simulink library "Generator_Lib_org"  (Simulink 10.0)
settings: Solver=ode45  StartTime=0.0  StopTime=10.0  RelTol=1e-3  EnableMultiTasking=on
undefined symbols (not defined in the file): radps2rpm, WT_Params
libraries: powerlib x12, fl_lib x10, nesl_utility x4, $bdroot x1, powerlib_extras x1
Description:
  | Copyright 2009-2017 The MathWorks, Inc. MathWorks, Inc.
settings Model: Creator=smiller  LastModifiedBy=bhisma

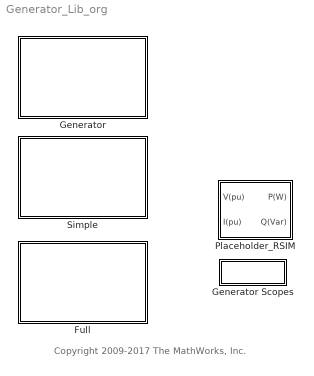
== system Generator_Lib_org ==
  note: Copyright 2009-2017 The MathWorks, Inc.
  Full : Subsystem
      mask Display:
      | image(imread('Generator_Full_IMAGE.jpg'));
      | port_label('LConn',1,'M');
      | port_label('LConn',2,'G');
      | port_label('RConn',1,'GrVa');
      | port_label('RConn',2,'GrVb');
      | port_label('RConn',3,'GrVc');
  Generator : Subsystem  BlockChoice=Full
      settings: TemplateBlock=self  MemberBlocks=Full,Simple
      mask Display: disp(' ')
  Generator Scopes : Subsystem
  Placeholder_RSIM : Subsystem
  Simple : Subsystem
      mask Display:
      | image(imread('Generator_Simple_IMAGE.jpg'));
      | port_label('LConn',1,'M');
      | port_label('LConn',2,'G');
      | port_label('RConn',1,'GrVa');
      | port_label('RConn',2,'GrVb');
      | port_label('RConn',3,'GrVc');

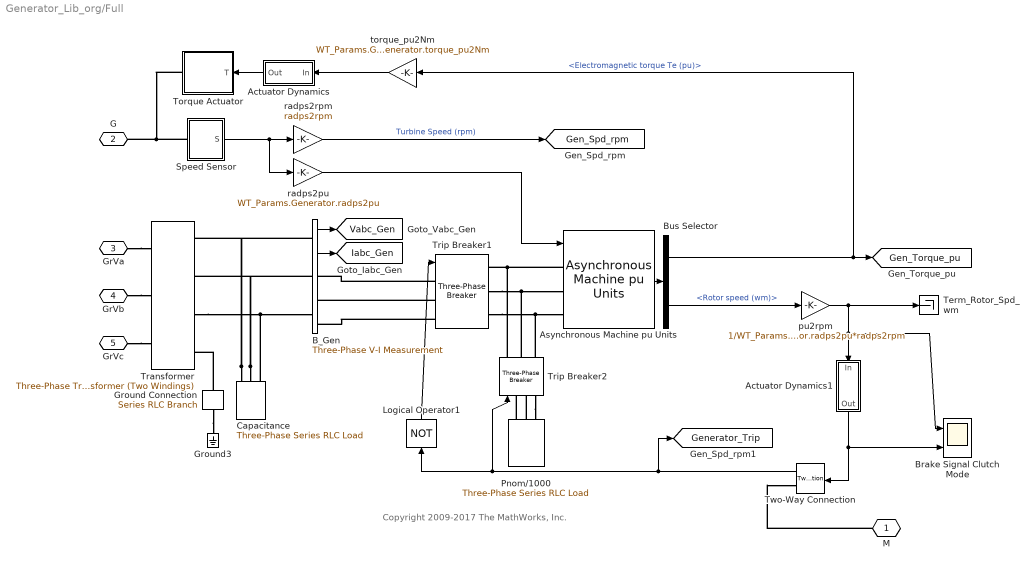
== system Generator_Lib_org/Full ==
  note: Copyright 2009-2017 The MathWorks, Inc.
  Actuator Dynamics : Subsystem  mask(First-order lag supporting vector signals){b=WT_Params.Generator.generator_time_constant, x_initial=0}
      mask prompts: b "Filter time constant"; x_initial "Initial output"
      mask help: Models a lag of the form 1/(b*s+1) where s is the Laplace operator.
  Actuator Dynamics1 : Subsystem  mask(First-order lag supporting vector signals){b=WT_Params.Generator.generator_time_constant, x_initial=0}
      mask prompts: b "Filter time constant"; x_initial "Initial output"
      mask help: Models a lag of the form 1/(b*s+1) where s is the Laplace operator.
  Asynchronous Machine pu Units : powerlib/Machines/Asynchronous Machine pu Units  RotorType=Squirrel-cage  PresetModel=No  MechanicalLoad=Speed w  ShowDetailedParameters=on  ReferenceFrame=Rotor  Units=pu  MeasurementBus=off  NominalParameters="[WT_Params.Generator.nominal_power  WT_Params.Generator.voltage WT_Params.Generator.frequency]"  Stator=[WT_Params.Generator.Stator.resistance WT_Params.Generator.Stator.inductance]  Rotor=[WT_Params.Generator.Rotor.resistance WT_Params.Generator.Rotor.inductance]  Cage1=[0.01909 0.0397]  Cage2=[0.01909 0.0397]  Lm=WT_Params.Generator.mutual_inductance  Mechanical=[0.09526 0.05479 3]  PolePairs=3  InitialConditions=[1 0 0 0 0 0 0 0]  SimulateSaturation=off  Saturation="[0.212,0.4201,0.8125,1.0979,1.4799,2.2457,3.2586,4.5763,6.4763 ;   0.5,0.7,0.9,1,1.1,1.2 ,1.3,1.4,1.5]"  LoadFlowParameters=1650000  TsPowergui=0  TsBlock=-1  IterativeModel=Forward Euler  IterativeDiscreteModel=Trapezoidal non iterative  Pmec=0
      settings: SourceProductName=Simscape Electrical  SourceProductBaseCode=PS
  B_Gen : powerlib/Measurements/Three-Phase V-I Measurement  VoltageMeasurement=phase-to-ground  SetLabelV=off  LabelV=Vabc  Vpu=on  VpuLL=off  CurrentMeasurement=yes  SetLabelI=off  LabelI=Iabc  Ipu=on  Pbase=WT_Params.Generator.nominal_power  Vbase=WT_Params.Generator.voltage  OutputType=Complex  PhasorSimulation=on  PSBequivalent=0
      settings: SourceProductName=Simscape Electrical
  Brake Signal Clutch Mode : Scope  NumInputPorts=2
  Bus Selector : BusSelector  OutputSignals=Mechanical.Electromagnetic torque Te (pu),Mechanical.Rotor speed (wm)
  Capacitance : powerlib/Elements/Three-Phase Series RLC Load  LConnTagsString=A|B|C  Configuration=Delta  NominalVoltage=WT_Params.Generator.voltage  Vabc=[1e3 1e3 1e3]  Vabcp=[1e3 1e3 1e3]  NominalFrequency=WT_Params.Generator.frequency  UnbalancedPower=off  ActivePower=0  InductivePower=0  CapacitivePower=200e3  Pabc=[10e3 9e3 11e3]  QLabc=[100 90 110]  QCabc=[100 90 110]  Pabcp=[10e3 9e3 11e3]  QLabcp=[100 90 110]  QCabcp=[100 90 110]  Measurements=None  LoadType=constant Z
      settings: SourceProductName=Simscape Electrical
  Ground Connection : powerlib/Elements/Series RLC Branch  LConnTagsString=__new0  RConnTagsString=__new0  BranchType=R  Resistance=10  Inductance=1.0  SetiL0=off  InitialCurrent=0  Capacitance=1.0  Setx0=off  InitialVoltage=0  Measurements=None
      settings: SourceProductName=Simscape Electrical
  Ground3 : powerlib/Elements/Ground  LConnTagsString=a
      settings: SourceProductName=Simscape Electrical
  Logical Operator1 : Logic  Operator=NOT  AllPortsSameDT=off  OutDataTypeStr=float('double')  SampleTime=0
  Pnom/1000 : powerlib/Elements/Three-Phase Series RLC Load  LConnTagsString=A|B|C  Configuration=Y (grounded)  NominalVoltage=WT_Params.Generator.voltage  Vabc=[1e3 1e3 1e3]  Vabcp=[1e3 1e3 1e3]  NominalFrequency=WT_Params.Generator.frequency  UnbalancedPower=off  ActivePower=WT_Params.Generator.nominal_power  InductivePower=0  CapacitivePower=0  Pabc=[10e3 9e3 11e3]  QLabc=[100 90 110]  QCabc=[100 90 110]  Pabcp=[10e3 9e3 11e3]  QLabcp=[100 90 110]  QCabcp=[100 90 110]  Measurements=None  LoadType=constant Z
      settings: SourceProductName=Simscape Electrical
  Speed Sensor : Subsystem
      mask Display:
      | plot([149.600878633536;150.016472378793;150.47508104106;150.972287968219;151.50330478576;152.063017511447;152.646035805762;153.246744883819;153.859359588817;154.477980106257;155.096648782383;155.709407499646;156.310355056631;156.893703999851;157.453836360095;157.985357756531;158.483149347555;158.942417128023;159.358738098149;159.728102859405;160.046954227227;160.312221488639;160.521349974904;160.672325664379;160.763694578642;160.794576785101;160.764674871227;160.674276808796;160.524253180566;160.316048796087;160.051668777399;159.733659248606;159.365082815313;158.949489070056;158.490880407788;157.993673480629;157.462656663088;156.908284800231], [156.971389291536;157.430657072004;157.84697804213;158.216342803387;158.535194171208;158.80046143262;159.009589918885;159.16056560836;159.251934522623;159.282816729083;159.252914815208;159.162516752777;159.012493124547;158.804288740068;158.53990872138;158.221899192587;157.853322759294;157.437729014037;156.979120351769;156.48191342461;155.950896607069;155.391183881382;154.808165587067;154.20745650901;153.594841804012;152.976221286573;152.357552610446;151.744793893183;151.143846336199;150.560497392978;150.000365032735;149.468843636298;148.971052045274;148.511784264806;148.095463294681;147.726098533424;147.407247165603;147.144199990631])
      | plot([152.057635404444;152.93604260309;153.834625296826;154.744729643097;155.657590839533;156.564417533794;157.45647648909;158.325176690034;159.162152078811;159.959342124889;160.709069452336;161.404113777147;162.037781442523;162.603969882449;163.097226392739;163.512800643557;163.846690427691;164.095680203997;164.257372064819;164.330208829146;164.313489039122;164.27939575172], [142.228020686971;141.979030910664;141.817339049842;141.744502285515;141.761222075539;141.867337399197;142.061826307913;142.342815767178;142.707599694895;143.152665022428;143.673725527376;144.265763112236;144.923076131425;145.639334301243;146.40763966397;147.220593018964;148.070365181011;148.948772379657;149.847355073393;150.757459419663;151.6703206161;152.055850472277])
      | plot([116.468514315784;116.438789536125;116.349901463023;116.202706137216;115.998621130155;115.739611892022;115.42817282337;115.067303252679;114.660478551187;114.211616663162;113.725040373958;113.205435679231;112.657806656235;112.087427271827;111.499790591278;110.900555877058;110.29549408704;109.690432297022;109.091197582803;108.503560902254;107.933181517846;107.38555249485;106.865947800123;106.379371510919;105.930509622894;105.523684921402;105.162815350711;104.851376282059;104.592367043926;104.388282036865;104.241086711057;104.152198637956;104.122473858297;104.152198637956;104.241086711057;104.388282036865;104.592367043926;104.851376282059;105.162815350711;105.523684921402;105.930509622894;106.379371510919;106.865947800123;107.38555249485;107.933181517846;108.503560902254;109.091197582803;109.690432297022;110.29549408704;110.900555877058;111.499790591278;112.087427271827;112.657806656235;113.205435679231;113.725040373958;114.211616663162;114.660478551187;115.067303252679;115.42817282337;115.739611892022;115.998621130155;116.202706137216;116.349901463023;116.438789536125;116.468514315784;116.468514315784], [111.618284136057;111.013222346039;110.413987631819;109.826350951271;109.255971566862;108.708342543866;108.188737849139;107.702161559936;107.253299671911;106.846474970419;106.485605399728;106.174166331075;105.915157092943;105.711072085881;105.563876760074;105.474988686973;105.445263907313;105.474988686973;105.563876760074;105.711072085881;105.915157092943;106.174166331075;106.485605399728;106.846474970419;107.253299671911;107.702161559936;108.188737849139;108.708342543866;109.255971566862;109.826350951271;110.413987631819;111.013222346039;111.618284136057;112.223345926075;112.822580640295;113.410217320843;113.980596705252;114.528225728247;115.047830422975;115.534406712178;115.983268600203;116.390093301695;116.750962872386;117.062401941038;117.321411179171;117.525496186232;117.67269151204;117.761579585141;117.7913043648;117.761579585141;117.67269151204;117.525496186232;117.321411179171;117.062401941038;116.750962872386;116.390093301695;115.983268600203;115.534406712178;115.047830422975;114.528225728247;113.980596705252;113.410217320843;112.822580640295;112.223345926075;111.618284136057;111.618284136057])
      | plot([239.23602886498;238.828071429858;237.608127977604;235.587947230552;232.78698463364;229.232214987837;224.957872668068;220.005121927465;214.421660463109;208.261260061133;201.583248745024;194.451939414329;186.936010476274;179.107844435155;171.042830809261;162.818640088593;154.514475725591;146.210311362589;137.986120641921;129.921107016027;122.092940974909;114.577012036853;107.445702706158;100.76769139005;94.607290988073;89.0238295237172;84.0710787831142;79.7967364633452;76.2419668175427;73.4410042206305;71.4208234735788;70.2008800213248;69.7929225862026;70.2008800213248;71.4208234735788;73.4410042206306;76.2419668175428;79.7967364633454;84.0710787831144;89.0238295237174;94.6072909880733;100.76769139005;107.445702706159;114.577012036853;122.092940974909;129.921107016027;137.986120641921;146.210311362589;154.514475725591;162.818640088593;171.042830809261;179.107844435155;186.936010476274;194.451939414329;201.583248745024;208.261260061133;214.421660463109;220.005121927465;224.957872668068;229.232214987837;232.78698463364;235.587947230552;237.608127977604;238.828071429858;239.23602886498;239.23602886498], [155.774275772274;147.47628550917;139.258209428443;131.199192095207;123.376846251889;115.866505365088;108.740498123116;102.067451871182;95.9116316925529;90.3323215006612;85.3832531026163;81.1120887325275;77.5599620381344;74.7610819412943;72.742403187363;71.5233667562631;71.1157126352191;71.5233667562631;72.742403187363;74.7610819412943;77.5599620381345;81.1120887325275;85.3832531026164;90.3323215006612;95.9116316925529;102.067451871182;108.740498123116;115.866505365089;123.376846251889;131.199192095207;139.258209428443;147.47628550917;155.774275772274;164.072266035377;172.290342116104;180.34935944934;188.171705292658;195.682046179459;202.808053421432;209.481099673365;215.636919851994;221.216230043886;226.165298441931;230.43646281202;233.988589506413;236.787469603253;238.806148357184;240.025184788284;240.432838909328;240.025184788284;238.806148357184;236.787469603253;233.988589506413;230.43646281202;226.165298441931;221.216230043886;215.636919851994;209.481099673365;202.808053421432;195.682046179459;188.171705292658;180.34935944934;172.290342116105;164.072266035378;155.774275772274;155.774275772274])
      | plot([252.715889364481;252.243022716633;250.828976737403;248.487369462568;245.240751850236;241.120390602797;236.165967051481;230.425195003451;223.953361231755;216.812793033479;209.072257983804;200.806301666664;192.094529760025;183.020841389688;173.672621134841;164.139897466795;154.514475725591;144.889053984387;135.356330316341;126.008110061494;116.934421691157;108.222649784518;99.9566934673787;92.2161584177032;85.075590219427;78.6037564477313;72.8629843997015;67.9085608483856;63.7881996009461;60.5415819886144;58.199974713779;56.7859287345493;56.3130620867014;56.7859287345493;58.1999747137791;60.5415819886146;63.7881996009463;67.9085608483858;72.8629843997018;78.6037564477315;85.0755902194273;92.2161584177035;99.9566934673791;108.222649784519;116.934421691157;126.008110061494;135.356330316341;144.889053984387;154.514475725591;164.139897466796;173.672621134841;183.020841389688;192.094529760025;200.806301666664;209.072257983803;216.812793033479;223.953361231755;230.425195003451;236.165967051481;241.120390602797;245.240751850236;248.487369462568;250.828976737403;252.243022716633;252.715889364481;252.715889364481], [154.514475725591;144.895228084285;135.36861905618;126.026395093992;116.958526921455;108.252343066071;99.9916888376535;92.2561188521535;85.1201308772245;78.6524483779929;72.9153586725213;67.9641130708855;63.8463947748555;60.6018596625959;58.2617543808809;56.8486154228053;56.3760520890355;56.8486154228053;58.2617543808809;60.6018596625959;63.8463947748555;67.9641130708856;72.9153586725213;78.652448377993;85.1201308772246;92.2561188521536;99.9916888376536;108.252343066072;116.958526921455;126.026395093992;135.36861905618;144.895228084285;154.514475725591;164.133723366898;173.660332395002;183.002556357191;192.070424529728;200.776608385111;209.037262613529;216.772832599029;223.908820573958;230.37650307319;236.113592778661;241.064838380297;245.182556676327;248.427091788587;250.767197070302;252.180336028377;252.652899362147;252.180336028377;250.767197070301;248.427091788587;245.182556676327;241.064838380297;236.113592778661;230.37650307319;223.908820573958;216.772832599029;209.037262613529;200.776608385111;192.070424529728;183.002556357191;173.660332395002;164.133723366898;154.514475725592;154.514475725591])
      | plot([154.514475725591;129.948374815285;179.017586633563;154.514475725591], [240.369848906994;203.583687543869;203.583687543869;240.369848906994])
      | plot([105.382273904979;149.60125554353], [115.271704271436;156.971085816622])
      | plot([144.688035361469;144.688035361469], [152.057865634561;203.583687543869])
      | plot([164.277926087379;164.277926087379], [152.057865634561;203.583687543869])
      | plot([159.112745895982;159.616665914655], [149.60125554353;149.60125554353])
      | plot([115.208714269102;159.364705905318], [107.901873998344;149.60125554353])
      | plot([0;311.800511553884;311.800511553884;0;0], [311.800511553884;311.800511553884;0;0;311.800511553884])
      | ;
      | color('red');
      | port_label('LConn', 1,'R')
      | port_label('output', 1,'W')
  Term_Rotor_Spd_wm : Terminator
  Torque Actuator : Subsystem
      mask Display:
      | plot([198.657636314574;187.5372000791;176.524559560751;165.725772507838;155.244837142898;145.182690602959;135.636236859729;126.697413481378;118.452306223496;110.980319976212;104.353414051689;98.6354091766174;93.8813728637222;90.1370890815176;87.4386173296598;85.811945366254;85.272738931537;85.8261908782356;87.4669711615554;90.1792781704262;93.9369909056548;98.7039205394262;104.434158933498;111.072520759669;118.555074964656;126.809760461083;135.75708011515;145.310866347487;155.379110974044;165.864851295207;176.667103899592;187.681837189509;192.988368326926], [283.691199740558;283.13774779386;281.49696751054;278.784660501669;275.026947766441;270.260018132669;264.529779738597;257.891417912426;250.40886370744;242.154178211013;233.206858556945;223.653072324609;213.584827698051;203.099087376889;192.296834772503;181.282101482586;170.160965409986;159.040529174513;148.027888656163;137.22910160325;126.748166238311;116.686019698372;107.139565955142;98.2007425767901;89.9556353189084;82.4836490716241;75.8567431471018;70.1387382720299;65.3847019591348;61.6404181769301;58.9419464250722;57.3152744616664;56.9214337615639])
      | plot([85.209725657478;1.11807254143059;1.11807254143059], [170.435198815539;170.435198815539;171.380048850551])
      | plot([283.691223012283;397.073227213696], [170.309218810871;170.309218810871])
      | plot([153.301918180659;255.34572196193], [170.309218810871;170.309218810871])
      | plot([198.654719861224;113.618216710165;198.654719861224], [85.2727156598121;170.309218810871;255.34572196193])
      | plot([198.654719861224;153.301918180659;198.654719861224], [215.662020491436;170.309218810871;124.956417130306])
      | plot([198.654719861224;283.691223012283;283.691223012283;187.316519441083;192.985619651154], [283.691223012283;283.691223012283;56.927214609459;56.927214609459;56.927214609459])
      | 
      | patch([395.419739652425;395.419739652425;5.6843418860808e-14;0;395.419739652425;394.947314634919;0.472425017505884;0.472425017505941;394.947314634919;394.947314634919;395.419739652425], [340.618437621742;5.6843418860808e-14;0;340.618437621742;340.618437621742;340.146012604237;340.146012604237;0.472425017505884;0.472425017505884;340.146012604237;340.618437621742], [1;1;1])
      | ;
      | color('red');
      | port_label('RConn', 1,'R')
      | port_label('Input', 1,'T')
  Transformer : powerlib/Elements/Three-Phase Transformer (Two Windings)  Winding1Connection=Yg  Winding2Connection=Yn  CoreType=Three single-phase transformers  SetSaturation=off  Hysteresis=off  DataFile='hysteresis'  SetInitialFlux=off  Measurements=None  UNITS=pu  NominalPower="[2e6  60]"  Winding1=[WT_Params.Grid.voltage, 0.025/30 , 0.025]  Winding2=[ WT_Params.Generator.voltage, 0.025/30 , 0.025]  Rm=500  Lm=inf  L0=0.5  Saturation=[ 0,0 ; 0.0024,1.2 ; 1.0,1.52 ]  InitialFluxes=[ 0.8 , -0.8 , 0.7 ]  BreakLoop=off  DiscreteSolver=Trapezoidal iterative  DataType=off  TransfoNumber=0
      settings: SourceProductName=Simscape Electrical
  Trip Breaker1 : powerlib/Elements/Three-Phase Breaker  InitialState=closed  SwitchA=on  SwitchB=on  SwitchC=on  SwitchTimes="[4/60  10/60]"  External=on  BreakerResistance=WT_Params.Generator.Breakers.ron  SnubberResistance=WT_Params.Generator.Breakers.rp  SnubberCapacitance=WT_Params.Generator.Breakers.cp  Measurements=None
      settings: SourceProductName=Simscape Electrical
  Trip Breaker2 : powerlib/Elements/Three-Phase Breaker  InitialState=open  SwitchA=on  SwitchB=on  SwitchC=on  SwitchTimes="[4/60  10/60]"  External=on  BreakerResistance=WT_Params.Generator.Breakers.ron  SnubberResistance=WT_Params.Generator.Breakers.rp  SnubberCapacitance=WT_Params.Generator.Breakers.cp  Measurements=None
      settings: SourceProductName=Simscape Electrical
  Two-Way Connection : TwoWayConnection
  pu2rpm : Gain  Gain=1/WT_Params.Generator.radps2pu*radps2rpm
  radps2pu : Gain  Gain=WT_Params.Generator.radps2pu
  radps2rpm : Gain  Gain=radps2rpm
  torque_pu2Nm : Gain  Gain=WT_Params.Generator.torque_pu2Nm
  M : PMIOPort  Tag=PMCPort  Side=Left
  G : PMIOPort  Port=2  Side=Left
  GrVa : PMIOPort  Port=3  Side=Right
  GrVb : PMIOPort  Port=4  Side=Right
  GrVc : PMIOPort  Port=5  Side=Right
  tag scope: Gen_Spd_rpm=global, Gen_Torque_pu=global, Generator_Trip=global, Iabc_Gen=global, Vabc_Gen=global
  wires:
  Logical Operator1/1 -> Trip Breaker1/1
  Two-Way Connection/1 -> Logical Operator1/1, Trip Breaker2/1, [Generator_Trip]
  pu2rpm/1 -> Brake Signal Clutch Mode/1, Actuator Dynamics1/1(In), Term_Rotor_Spd_wm/1
  Bus Selector/2 -> pu2rpm/1  "<Rotor speed (wm)>"
  radps2rpm/1 -> [Gen_Spd_rpm]  "Turbine Speed (rpm)"
  torque_pu2Nm/1 -> Actuator Dynamics/1(In)
  radps2pu/1 -> Asynchronous Machine pu Units/1
  Bus Selector/1 -> [Gen_Torque_pu], torque_pu2Nm/1  "<Electromagnetic torque Te (pu)>"
  Speed Sensor/1(S) -> radps2pu/1, radps2rpm/1
  Asynchronous Machine pu Units/1 -> Bus Selector/1
  B_Gen/1 -> [Vabc_Gen]
  B_Gen/2 -> [Iabc_Gen]
  Actuator Dynamics/1(Out) -> Torque Actuator/1(T)
  Actuator Dynamics1/1(Out) -> Brake Signal Clutch Mode/2, Two-Way Connection/1
  connections:
  Trip Breaker1/LConn1 -- B_Gen/RConn1
  Trip Breaker1/LConn2 -- B_Gen/RConn2
  Trip Breaker1/LConn3 -- B_Gen/RConn3
  Trip Breaker2/RConn1 -- Trip Breaker1/RConn1 -- Asynchronous Machine pu Units/LConn1
  Trip Breaker2/RConn2 -- Asynchronous Machine pu Units/LConn2 -- Trip Breaker1/RConn2
  Trip Breaker2/RConn3 -- Asynchronous Machine pu Units/LConn3 -- Trip Breaker1/RConn3
  Pnom/1000/LConn2 -- Trip Breaker2/LConn2
  Trip Breaker2/LConn3 -- Pnom/1000/LConn3
  Pnom/1000/LConn1 -- Trip Breaker2/LConn1
  Ground Connection/LConn1 -- Transformer/RConn4
  Ground Connection/RConn1 -- Ground3/LConn1
  GrVa/RConn1 -- Transformer/LConn1
  GrVc/RConn1 -- Transformer/LConn3
  GrVb/RConn1 -- Transformer/LConn2
  Torque Actuator/RConn1 -- G/RConn1 -- Speed Sensor/LConn1
  Capacitance/LConn3 -- B_Gen/LConn3 -- Transformer/RConn3
  Capacitance/LConn1 -- B_Gen/LConn1 -- Transformer/RConn1
  M/RConn1 -- Two-Way Connection/RConn1
  Capacitance/LConn2 -- B_Gen/LConn2 -- Transformer/RConn2

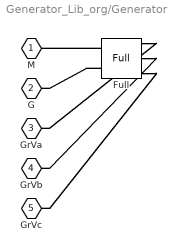
== system Generator_Lib_org/Generator ==
  Full : $bdroot/Full  SystemSampleTime=-1  Latency=0  AutoFrameSizeCalculation=off
  M : PMIOPort  Side=Left
  G : PMIOPort  Port=2  Side=Left
  GrVa : PMIOPort  Port=3  Side=Right
  GrVb : PMIOPort  Port=4  Side=Right
  GrVc : PMIOPort  Port=5  Side=Right
  connections:
  Full/LConn1 -- M/RConn1
  Full/LConn2 -- G/RConn1
  Full/RConn1 -- GrVa/RConn1
  Full/RConn2 -- GrVb/RConn1
  Full/RConn3 -- GrVc/RConn1

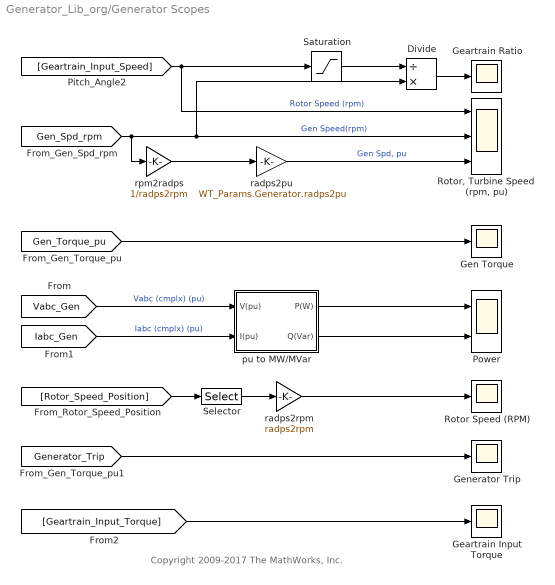
== system Generator_Lib_org/Generator Scopes ==
  note: Copyright 2009-2017 The MathWorks, Inc.
  Divide : Product  Inputs=/*
  Geartrain Input Torque : Scope
  Geartrain Ratio : Scope
  Gen Torque : Scope
  Generator Trip : Scope
  Power : Scope  NumInputPorts=2
  Rotor Speed (RPM) : Scope
  "Rotor, Turbine Speed  (rpm, pu)" : Scope  NumInputPorts=3
  Saturation : Saturate  UpperLimit=inf  LowerLimit=eps
  Selector : Selector  InputPortWidth=2  IndexOptions=Index vector (dialog)  Indices=[2]  OutputSizes=1
  pu to MW/MVar : Subsystem
  radps2pu : Gain  Gain=WT_Params.Generator.radps2pu
  radps2rpm : Gain  Gain=radps2rpm
  rpm2radps : Gain  Gain=1/radps2rpm
  wires:
  [Geartrain_Input_Torque] -> Geartrain Input Torque/1
  Saturation/1 -> Divide/1
  radps2rpm/1 -> Rotor Speed (RPM)/1
  Selector/1 -> radps2rpm/1
  [Rotor_Speed_Position] -> Selector/1
  [Gen_Spd_rpm] -> rpm2radps/1, Divide/2, "Rotor, Turbine Speed  (rpm, pu)"/2  "Gen Speed(rpm)"
  Divide/1 -> Geartrain Ratio/1
  rpm2radps/1 -> radps2pu/1
  radps2pu/1 -> "Rotor, Turbine Speed  (rpm, pu)"/3  "Gen Spd, pu"
  [Geartrain_Input_Speed] -> Saturation/1, "Rotor, Turbine Speed  (rpm, pu)"/1  "Rotor Speed (rpm)"
  [Vabc_Gen] -> pu to MW/MVar/1(V(pu))  "Vabc (cmplx) (pu)"
  [Iabc_Gen] -> pu to MW/MVar/2(I(pu))  "Iabc (cmplx) (pu)"
  [Gen_Torque_pu] -> Gen Torque/1
  pu to MW/MVar/1(P(W)) -> Power/1
  pu to MW/MVar/2(Q(Var)) -> Power/2
  [Generator_Trip] -> Generator Trip/1

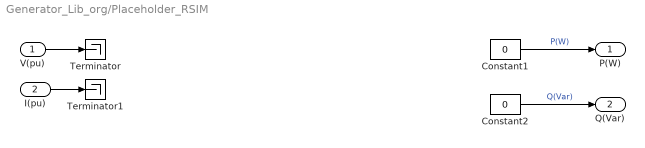
== system Generator_Lib_org/Placeholder_RSIM ==
  V(pu) : Inport
  I(pu) : Inport  Port=2
  Constant1 : Constant  Value=0
  Constant2 : Constant  Value=0
  Terminator : Terminator
  Terminator1 : Terminator
  P(W) : Outport
  Q(Var) : Outport  Port=2
  wires:
  Constant2/1 -> Q(Var)/1  "Q(Var)"
  Constant1/1 -> P(W)/1  "P(W)"
  I(pu)/1 -> Terminator1/1
  V(pu)/1 -> Terminator/1

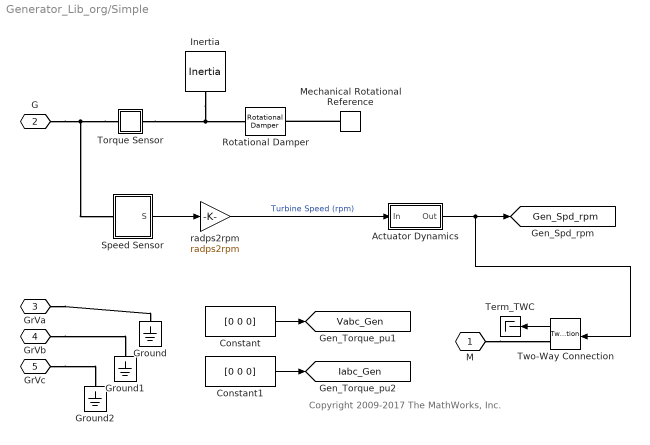
== system Generator_Lib_org/Simple ==
  note: Copyright 2009-2017 The MathWorks, Inc.
  Actuator Dynamics : Subsystem  mask(First-order lag supporting vector signals){b=WT_Params.Generator.generator_time_constant, x_initial=0}
      mask prompts: b "Filter time constant"; x_initial "Initial output"
      mask help: Models a lag of the form 1/(b*s+1) where s is the Laplace operator.
  Constant : Constant  Value=[0 0 0]  OutDataTypeStr=Inherit: Inherit via back propagation
  Constant1 : Constant  Value=[0 0 0]  OutDataTypeStr=Inherit: Inherit via back propagation
  Ground : powerlib/Elements/Ground  LConnTagsString=a
      settings: SourceProductName=Simscape Electrical
  Ground1 : powerlib/Elements/Ground  LConnTagsString=a
      settings: SourceProductName=Simscape Electrical
  Ground2 : powerlib/Elements/Ground  LConnTagsString=a
      settings: SourceProductName=Simscape Electrical
  Inertia : fl_lib/Mechanical/Rotational Elements/Inertia  inertia=WT_Params.Generator.Simple.inertia kg*m^2  w_specify=on  w_priority=High  w=0 rad/s  w_nominal_specify=off  w_nominal_unit=rad/s  w_nominal_value=1  t_specify=off  t_priority=High  t=0 N*m  t_nominal_specify=off  t_nominal_unit=N*m  t_nominal_value=1
  Mechanical Rotational Reference : fl_lib/Mechanical/Rotational Elements/Mechanical Rotational Reference
  Rotational Damper : fl_lib/Mechanical/Rotational Elements/Rotational Damper  D=WT_Params.Generator.Simple.damping N*m/(rad/s)  w_specify=off  w_priority=High  w=0 rad/s  w_nominal_specify=off  w_nominal_unit=rad/s  w_nominal_value=1  t_specify=off  t_priority=High  t=0 N*m  t_nominal_specify=off  t_nominal_unit=N*m  t_nominal_value=1
  Speed Sensor : Subsystem
      mask Display:
      | plot([149.600878633536;150.016472378793;150.47508104106;150.972287968219;151.50330478576;152.063017511447;152.646035805762;153.246744883819;153.859359588817;154.477980106257;155.096648782383;155.709407499646;156.310355056631;156.893703999851;157.453836360095;157.985357756531;158.483149347555;158.942417128023;159.358738098149;159.728102859405;160.046954227227;160.312221488639;160.521349974904;160.672325664379;160.763694578642;160.794576785101;160.764674871227;160.674276808796;160.524253180566;160.316048796087;160.051668777399;159.733659248606;159.365082815313;158.949489070056;158.490880407788;157.993673480629;157.462656663088;156.908284800231], [156.971389291536;157.430657072004;157.84697804213;158.216342803387;158.535194171208;158.80046143262;159.009589918885;159.16056560836;159.251934522623;159.282816729083;159.252914815208;159.162516752777;159.012493124547;158.804288740068;158.53990872138;158.221899192587;157.853322759294;157.437729014037;156.979120351769;156.48191342461;155.950896607069;155.391183881382;154.808165587067;154.20745650901;153.594841804012;152.976221286573;152.357552610446;151.744793893183;151.143846336199;150.560497392978;150.000365032735;149.468843636298;148.971052045274;148.511784264806;148.095463294681;147.726098533424;147.407247165603;147.144199990631])
      | plot([152.057635404444;152.93604260309;153.834625296826;154.744729643097;155.657590839533;156.564417533794;157.45647648909;158.325176690034;159.162152078811;159.959342124889;160.709069452336;161.404113777147;162.037781442523;162.603969882449;163.097226392739;163.512800643557;163.846690427691;164.095680203997;164.257372064819;164.330208829146;164.313489039122;164.27939575172], [142.228020686971;141.979030910664;141.817339049842;141.744502285515;141.761222075539;141.867337399197;142.061826307913;142.342815767178;142.707599694895;143.152665022428;143.673725527376;144.265763112236;144.923076131425;145.639334301243;146.40763966397;147.220593018964;148.070365181011;148.948772379657;149.847355073393;150.757459419663;151.6703206161;152.055850472277])
      | plot([116.468514315784;116.438789536125;116.349901463023;116.202706137216;115.998621130155;115.739611892022;115.42817282337;115.067303252679;114.660478551187;114.211616663162;113.725040373958;113.205435679231;112.657806656235;112.087427271827;111.499790591278;110.900555877058;110.29549408704;109.690432297022;109.091197582803;108.503560902254;107.933181517846;107.38555249485;106.865947800123;106.379371510919;105.930509622894;105.523684921402;105.162815350711;104.851376282059;104.592367043926;104.388282036865;104.241086711057;104.152198637956;104.122473858297;104.152198637956;104.241086711057;104.388282036865;104.592367043926;104.851376282059;105.162815350711;105.523684921402;105.930509622894;106.379371510919;106.865947800123;107.38555249485;107.933181517846;108.503560902254;109.091197582803;109.690432297022;110.29549408704;110.900555877058;111.499790591278;112.087427271827;112.657806656235;113.205435679231;113.725040373958;114.211616663162;114.660478551187;115.067303252679;115.42817282337;115.739611892022;115.998621130155;116.202706137216;116.349901463023;116.438789536125;116.468514315784;116.468514315784], [111.618284136057;111.013222346039;110.413987631819;109.826350951271;109.255971566862;108.708342543866;108.188737849139;107.702161559936;107.253299671911;106.846474970419;106.485605399728;106.174166331075;105.915157092943;105.711072085881;105.563876760074;105.474988686973;105.445263907313;105.474988686973;105.563876760074;105.711072085881;105.915157092943;106.174166331075;106.485605399728;106.846474970419;107.253299671911;107.702161559936;108.188737849139;108.708342543866;109.255971566862;109.826350951271;110.413987631819;111.013222346039;111.618284136057;112.223345926075;112.822580640295;113.410217320843;113.980596705252;114.528225728247;115.047830422975;115.534406712178;115.983268600203;116.390093301695;116.750962872386;117.062401941038;117.321411179171;117.525496186232;117.67269151204;117.761579585141;117.7913043648;117.761579585141;117.67269151204;117.525496186232;117.321411179171;117.062401941038;116.750962872386;116.390093301695;115.983268600203;115.534406712178;115.047830422975;114.528225728247;113.980596705252;113.410217320843;112.822580640295;112.223345926075;111.618284136057;111.618284136057])
      | plot([239.23602886498;238.828071429858;237.608127977604;235.587947230552;232.78698463364;229.232214987837;224.957872668068;220.005121927465;214.421660463109;208.261260061133;201.583248745024;194.451939414329;186.936010476274;179.107844435155;171.042830809261;162.818640088593;154.514475725591;146.210311362589;137.986120641921;129.921107016027;122.092940974909;114.577012036853;107.445702706158;100.76769139005;94.607290988073;89.0238295237172;84.0710787831142;79.7967364633452;76.2419668175427;73.4410042206305;71.4208234735788;70.2008800213248;69.7929225862026;70.2008800213248;71.4208234735788;73.4410042206306;76.2419668175428;79.7967364633454;84.0710787831144;89.0238295237174;94.6072909880733;100.76769139005;107.445702706159;114.577012036853;122.092940974909;129.921107016027;137.986120641921;146.210311362589;154.514475725591;162.818640088593;171.042830809261;179.107844435155;186.936010476274;194.451939414329;201.583248745024;208.261260061133;214.421660463109;220.005121927465;224.957872668068;229.232214987837;232.78698463364;235.587947230552;237.608127977604;238.828071429858;239.23602886498;239.23602886498], [155.774275772274;147.47628550917;139.258209428443;131.199192095207;123.376846251889;115.866505365088;108.740498123116;102.067451871182;95.9116316925529;90.3323215006612;85.3832531026163;81.1120887325275;77.5599620381344;74.7610819412943;72.742403187363;71.5233667562631;71.1157126352191;71.5233667562631;72.742403187363;74.7610819412943;77.5599620381345;81.1120887325275;85.3832531026164;90.3323215006612;95.9116316925529;102.067451871182;108.740498123116;115.866505365089;123.376846251889;131.199192095207;139.258209428443;147.47628550917;155.774275772274;164.072266035377;172.290342116104;180.34935944934;188.171705292658;195.682046179459;202.808053421432;209.481099673365;215.636919851994;221.216230043886;226.165298441931;230.43646281202;233.988589506413;236.787469603253;238.806148357184;240.025184788284;240.432838909328;240.025184788284;238.806148357184;236.787469603253;233.988589506413;230.43646281202;226.165298441931;221.216230043886;215.636919851994;209.481099673365;202.808053421432;195.682046179459;188.171705292658;180.34935944934;172.290342116105;164.072266035378;155.774275772274;155.774275772274])
      | plot([252.715889364481;252.243022716633;250.828976737403;248.487369462568;245.240751850236;241.120390602797;236.165967051481;230.425195003451;223.953361231755;216.812793033479;209.072257983804;200.806301666664;192.094529760025;183.020841389688;173.672621134841;164.139897466795;154.514475725591;144.889053984387;135.356330316341;126.008110061494;116.934421691157;108.222649784518;99.9566934673787;92.2161584177032;85.075590219427;78.6037564477313;72.8629843997015;67.9085608483856;63.7881996009461;60.5415819886144;58.199974713779;56.7859287345493;56.3130620867014;56.7859287345493;58.1999747137791;60.5415819886146;63.7881996009463;67.9085608483858;72.8629843997018;78.6037564477315;85.0755902194273;92.2161584177035;99.9566934673791;108.222649784519;116.934421691157;126.008110061494;135.356330316341;144.889053984387;154.514475725591;164.139897466796;173.672621134841;183.020841389688;192.094529760025;200.806301666664;209.072257983803;216.812793033479;223.953361231755;230.425195003451;236.165967051481;241.120390602797;245.240751850236;248.487369462568;250.828976737403;252.243022716633;252.715889364481;252.715889364481], [154.514475725591;144.895228084285;135.36861905618;126.026395093992;116.958526921455;108.252343066071;99.9916888376535;92.2561188521535;85.1201308772245;78.6524483779929;72.9153586725213;67.9641130708855;63.8463947748555;60.6018596625959;58.2617543808809;56.8486154228053;56.3760520890355;56.8486154228053;58.2617543808809;60.6018596625959;63.8463947748555;67.9641130708856;72.9153586725213;78.652448377993;85.1201308772246;92.2561188521536;99.9916888376536;108.252343066072;116.958526921455;126.026395093992;135.36861905618;144.895228084285;154.514475725591;164.133723366898;173.660332395002;183.002556357191;192.070424529728;200.776608385111;209.037262613529;216.772832599029;223.908820573958;230.37650307319;236.113592778661;241.064838380297;245.182556676327;248.427091788587;250.767197070302;252.180336028377;252.652899362147;252.180336028377;250.767197070301;248.427091788587;245.182556676327;241.064838380297;236.113592778661;230.37650307319;223.908820573958;216.772832599029;209.037262613529;200.776608385111;192.070424529728;183.002556357191;173.660332395002;164.133723366898;154.514475725592;154.514475725591])
      | plot([154.514475725591;129.948374815285;179.017586633563;154.514475725591], [240.369848906994;203.583687543869;203.583687543869;240.369848906994])
      | plot([105.382273904979;149.60125554353], [115.271704271436;156.971085816622])
      | plot([144.688035361469;144.688035361469], [152.057865634561;203.583687543869])
      | plot([164.277926087379;164.277926087379], [152.057865634561;203.583687543869])
      | plot([159.112745895982;159.616665914655], [149.60125554353;149.60125554353])
      | plot([115.208714269102;159.364705905318], [107.901873998344;149.60125554353])
      | plot([0;311.800511553884;311.800511553884;0;0], [311.800511553884;311.800511553884;0;0;311.800511553884])
      | ;
      | color('red');
      | port_label('LConn', 1,'R')
      | port_label('output', 1,'W')
  Term_TWC : Terminator
  Torque Sensor : Subsystem
      mask Display: disp('S');
  Two-Way Connection : TwoWayConnection
  radps2rpm : Gain  Gain=radps2rpm
  M : PMIOPort  Tag=PMCPort  Side=Left
  G : PMIOPort  Port=2  Side=Left
  GrVa : PMIOPort  Port=3  Side=Right
  GrVb : PMIOPort  Port=4  Side=Right
  GrVc : PMIOPort  Port=5  Side=Right
  tag scope: Gen_Spd_rpm=global, Iabc_Gen=global, Vabc_Gen=global
  wires:
  Constant1/1 -> [Iabc_Gen]
  Constant/1 -> [Vabc_Gen]
  Speed Sensor/1(S) -> radps2rpm/1
  radps2rpm/1 -> Actuator Dynamics/1(In)  "Turbine Speed (rpm)"
  Two-Way Connection/1 -> Term_TWC/1
  Actuator Dynamics/1(Out) -> Two-Way Connection/1, [Gen_Spd_rpm]
  connections:
  M/RConn1 -- Two-Way Connection/RConn1
  Torque Sensor/LConn1 -- G/RConn1 -- Speed Sensor/LConn1
  GrVb/RConn1 -- Ground1/LConn1
  GrVc/RConn1 -- Ground2/LConn1
  GrVa/RConn1 -- Ground/LConn1
  Mechanical Rotational Reference/LConn1 -- Rotational Damper/RConn1
  Torque Sensor/RConn1 -- Inertia/LConn1 -- Rotational Damper/LConn1

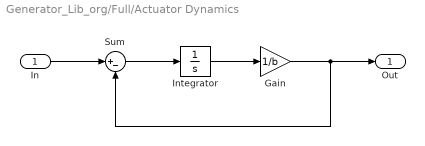
== system Generator_Lib_org/Full/Actuator Dynamics ==
  In : Inport
  Gain : Gain  Gain=1/b
  Integrator : Integrator  InitialCondition=x_initial
  Sum : Sum  Inputs=|+-  SaturateOnIntegerOverflow=on  InputSameDT=on  OutDataTypeStr=Inherit: Same as first input
  Out : Outport
  wires:
  Gain/1 -> Out/1, Sum/2
  Integrator/1 -> Gain/1
  In/1 -> Sum/1
  Sum/1 -> Integrator/1

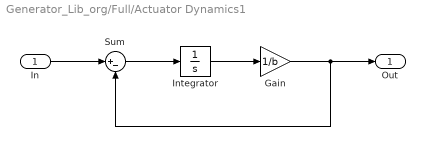
== system Generator_Lib_org/Full/Actuator Dynamics1 ==
  In : Inport
  Gain : Gain  Gain=1/b
  Integrator : Integrator  InitialCondition=x_initial
  Sum : Sum  Inputs=|+-  SaturateOnIntegerOverflow=on  InputSameDT=on  OutDataTypeStr=Inherit: Same as first input
  Out : Outport
  wires:
  Sum/1 -> Integrator/1
  In/1 -> Sum/1
  Integrator/1 -> Gain/1
  Gain/1 -> Sum/2, Out/1

== system Generator_Lib_org/Full/Speed Sensor ==
  Ideal Rotational Motion Sensor : fl_lib/Mechanical/Mechanical Sensors/Ideal Rotational Motion Sensor  offset=0 rad
  Mechanical Rotational Reference1 : fl_lib/Mechanical/Rotational Elements/Mechanical Rotational Reference
  PS-Simulink Converter : nesl_utility/PS-Simulink Converter  PhysicalDomain=network_engine_domain  SubClassName=ps_output  LeftPortType=input  RightPortType=output  PseudoPeriodic=off  Frequencies=[]  Unit=rad/s  AffineConversion=off
  R : PMIOPort  Side=Left
  S : Outport
  wires:
  PS-Simulink Converter/1 -> S/1
  connections:
  Ideal Rotational Motion Sensor/RConn2 -- PS-Simulink Converter/LConn1
  R/RConn1 -- Ideal Rotational Motion Sensor/LConn1
  Mechanical Rotational Reference1/LConn1 -- Ideal Rotational Motion Sensor/RConn1

== system Generator_Lib_org/Full/Torque Actuator ==
  T : Inport
  Ideal Torque Source : fl_lib/Mechanical/Mechanical Sources/Ideal Torque Source
  Mechanical Rotational Reference : fl_lib/Mechanical/Rotational Elements/Mechanical Rotational Reference
  Simulink-PS Converter : nesl_utility/Simulink-PS Converter  PhysicalDomain=network_engine_domain  SubClassName=ps_input  LeftPortType=input  RightPortType=output  PseudoPeriodic=off  Frequencies=[]  NoiseDistribution=none  NoiseParameters=[]  Unit=1  AffineConversion=off  FilteringAndDerivatives=filter  SimscapeFilterOrder=1  InputFilterTimeConstant=WT_Params.Generator.PSLD_Interface_Filter_Coeff  UdotUserProvided=1
  R : PMIOPort  Side=Right
  wires:
  T/1 -> Simulink-PS Converter/1
  connections:
  Simulink-PS Converter/RConn1 -- Ideal Torque Source/RConn1
  Mechanical Rotational Reference/LConn1 -- Ideal Torque Source/RConn2
  R/RConn1 -- Ideal Torque Source/LConn1

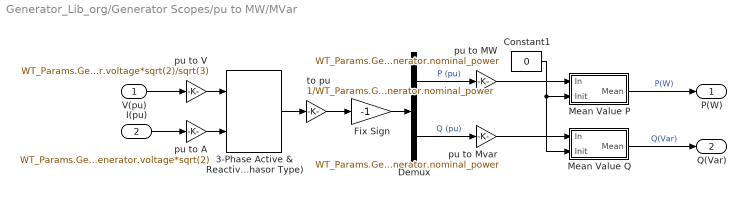
== system Generator_Lib_org/Generator Scopes/pu to MW/MVar ==
  V(pu) : Inport
  I(pu) : Inport  Port=2
  3-Phase Active & Reactive Power (Phasor Type) : powerlib_extras/Phasor Library/3-Phase Active & Reactive Power (Phasor Type)
      settings: SourceProductName=Simscape Electrical  SourceProductBaseCode=PS
  Constant1 : Constant  Value=0
  Demux : Demux  Outputs=2
  Fix Sign : Gain  Gain=-1  SaturateOnIntegerOverflow=on  OutDataTypeStr=Inherit: Same as input  ParamDataTypeStr=Inherit: Same as input
  Mean Value P : Subsystem  mask(Mean value){Period=1/WT_Params.Generator.frequency}
      mask prompts: Period "Averaging period (s):"
      mask help: This block uses the running window averaging technique to compute the mean value of the input signal over the specified period.
  Mean Value Q : Subsystem  mask(Mean value){Period=1/WT_Params.Generator.frequency}
      mask prompts: Period "Averaging period (s):"
      mask help: This block uses the running window averaging technique to compute the mean value of the input signal over the specified period.
  pu to A : Gain  Gain=WT_Params.Generator.nominal_power/sqrt(3)/WT_Params.Generator.voltage*sqrt(2)  SaturateOnIntegerOverflow=on  OutDataTypeStr=Inherit: Same as input  ParamDataTypeStr=Inherit: Same as input
  pu to MW : Gain  Gain=WT_Params.Generator.nominal_power  SaturateOnIntegerOverflow=on  OutDataTypeStr=Inherit: Same as input  ParamDataTypeStr=Inherit: Same as input
  pu to Mvar : Gain  Gain=WT_Params.Generator.nominal_power  SaturateOnIntegerOverflow=on  OutDataTypeStr=Inherit: Same as input  ParamDataTypeStr=Inherit: Same as input
  pu to V : Gain  Gain=WT_Params.Generator.voltage*sqrt(2)/sqrt(3)  SaturateOnIntegerOverflow=on  OutDataTypeStr=Inherit: Same as input  ParamDataTypeStr=Inherit: Same as input
  to pu : Gain  Gain=1/WT_Params.Generator.nominal_power  SaturateOnIntegerOverflow=on  OutDataTypeStr=Inherit: Same as input  ParamDataTypeStr=Inherit: Same as input
  P(W) : Outport
  Q(Var) : Outport  Port=2
  wires:
  Demux/1 -> pu to MW/1  "P (pu)"
  Demux/2 -> pu to Mvar/1  "Q (pu)"
  pu to V/1 -> 3-Phase Active & Reactive Power (Phasor Type)/1
  3-Phase Active & Reactive Power (Phasor Type)/1 -> to pu/1
  to pu/1 -> Fix Sign/1
  Fix Sign/1 -> Demux/1
  pu to A/1 -> 3-Phase Active & Reactive Power (Phasor Type)/2
  pu to MW/1 -> Mean Value P/1(In)
  Constant1/1 -> Mean Value P/2(Init), Mean Value Q/2(Init)
  pu to Mvar/1 -> Mean Value Q/1(In)
  V(pu)/1 -> pu to V/1
  I(pu)/1 -> pu to A/1
  Mean Value P/1(Mean) -> P(W)/1  "P(W)"
  Mean Value Q/1(Mean) -> Q(Var)/1  "Q(Var)"

== system Generator_Lib_org/Simple/Actuator Dynamics ==
  In : Inport
  Gain : Gain  Gain=1/b
  Integrator : Integrator  InitialCondition=x_initial
  Sum : Sum  Inputs=|+-  SaturateOnIntegerOverflow=on  InputSameDT=on  OutDataTypeStr=Inherit: Same as first input
  Out : Outport
  wires:
  Sum/1 -> Integrator/1
  In/1 -> Sum/1
  Integrator/1 -> Gain/1
  Gain/1 -> Sum/2, Out/1

== system Generator_Lib_org/Simple/Speed Sensor ==
  Ideal Rotational Motion Sensor : fl_lib/Mechanical/Mechanical Sensors/Ideal Rotational Motion Sensor  offset=0 rad
  Mechanical Rotational Reference1 : fl_lib/Mechanical/Rotational Elements/Mechanical Rotational Reference
  PS-Simulink Converter : nesl_utility/PS-Simulink Converter  PhysicalDomain=network_engine_domain  SubClassName=ps_output  LeftPortType=input  RightPortType=output  PseudoPeriodic=off  Frequencies=[]  Unit=1  AffineConversion=off
  R : PMIOPort  Side=Left
  S : Outport
  wires:
  PS-Simulink Converter/1 -> S/1
  connections:
  Mechanical Rotational Reference1/LConn1 -- Ideal Rotational Motion Sensor/RConn1
  R/RConn1 -- Ideal Rotational Motion Sensor/LConn1
  Ideal Rotational Motion Sensor/RConn2 -- PS-Simulink Converter/LConn1

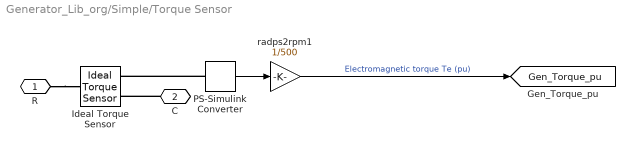
== system Generator_Lib_org/Simple/Torque Sensor ==
  Ideal Torque Sensor : fl_lib/Mechanical/Mechanical Sensors/Ideal Torque Sensor
  PS-Simulink Converter : nesl_utility/PS-Simulink Converter  PhysicalDomain=network_engine_domain  SubClassName=ps_output  LeftPortType=input  RightPortType=output  PseudoPeriodic=off  Frequencies=[]  Unit=1  AffineConversion=off
  radps2rpm1 : Gain  Gain=1/500
  R : PMIOPort  Side=Left
  C : PMIOPort  Port=2  Side=Right
  tag scope: Gen_Torque_pu=global
  wires:
  PS-Simulink Converter/1 -> radps2rpm1/1
  radps2rpm1/1 -> [Gen_Torque_pu]  "Electromagnetic torque Te (pu)"
  connections:
  R/RConn1 -- Ideal Torque Sensor/LConn1
  C/RConn1 -- Ideal Torque Sensor/RConn1
  PS-Simulink Converter/LConn1 -- Ideal Torque Sensor/RConn2

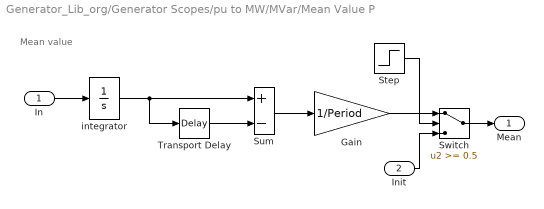
== system Generator_Lib_org/Generator Scopes/pu to MW/MVar/Mean Value P ==
  note: Mean value
  In : Inport
  Init : Inport  Port=2
  Gain : Gain  Gain=1/Period  SaturateOnIntegerOverflow=on  OutDataTypeStr=Inherit: Same as input  ParamDataTypeStr=Inherit: Same as input
  Step : Step  Time=Period+eps  SampleTime=0
  Sum : Sum  Inputs=+-  SaturateOnIntegerOverflow=on  InputSameDT=on  OutDataTypeStr=Inherit: Same as first input
  Switch : Switch  Threshold=0.5  SaturateOnIntegerOverflow=on
  Transport Delay : TransportDelay  DelayTime=Period
  integrator : Integrator
  Mean : Outport
  wires:
  Init/1 -> Switch/3
  Step/1 -> Switch/2
  Switch/1 -> Mean/1
  Gain/1 -> Switch/1
  Sum/1 -> Gain/1
  In/1 -> integrator/1
  integrator/1 -> Sum/1, Transport Delay/1
  Transport Delay/1 -> Sum/2

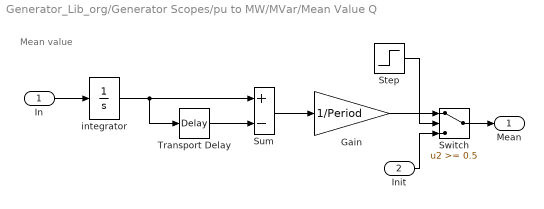
== system Generator_Lib_org/Generator Scopes/pu to MW/MVar/Mean Value Q ==
  note: Mean value
  In : Inport
  Init : Inport  Port=2
  Gain : Gain  Gain=1/Period  SaturateOnIntegerOverflow=on  OutDataTypeStr=Inherit: Same as input  ParamDataTypeStr=Inherit: Same as input
  Step : Step  Time=Period+eps  SampleTime=0
  Sum : Sum  Inputs=+-  SaturateOnIntegerOverflow=on  InputSameDT=on  OutDataTypeStr=Inherit: Same as first input
  Switch : Switch  Threshold=0.5  SaturateOnIntegerOverflow=on
  Transport Delay : TransportDelay  DelayTime=Period
  integrator : Integrator
  Mean : Outport
  wires:
  Transport Delay/1 -> Sum/2
  integrator/1 -> Transport Delay/1, Sum/1
  In/1 -> integrator/1
  Sum/1 -> Gain/1
  Gain/1 -> Switch/1
  Switch/1 -> Mean/1
  Step/1 -> Switch/2
  Init/1 -> Switch/3
